simulink model "BMS_PIL_Wrapper"  (R2025b)
settings: Solver=ode3  StartTime=0.0  StopTime=20  FixedStep=.001  MaxStep=.01  RelTol=1e-3  EnableMultiTasking=on
PreLoadFcn:
  | setup_pil;
InitFcn:
  | battery_init;
  | Full_Charge_Volt=4.2; % unit volts
  | Cutoff_Volt=3; % unit volts
  | Delta=.02;
  | ContactorTime=20;
  | ContactorTimeOut=100;
  | High_TempLim=333;
  | Low_TempLim=253;
  | Sensor_Fault_Treshold=.02;
  | CurrentTimeout=1;
  | Allowed_Delta=.04;
  | Bal_On_Time=30;
  | Bal_Off_Time=5;
  | BalNotAct_Time=10;
values from neighbouring files (symbols this model uses):
  Cell_Num = 12    [From_Plant_IC.m]
  Fly_Cycle_Current = [ ... (first row only)    [battery_init.m]
undefined symbols (not defined in the file or in its folder): SRE
libraries: fl_lib x69, nesl_utility x54, ee_lib x12, batteryecm_lib x12, simulink x5, BatteryCurrentManagement x1
(part 4 of 4)

== stateflow chart BMS_PIL_Wrapper/Test Sequence ==
  state Flying
    State_Required=SRE.Charge
  state step_2
  (default) -> Flying
  Flying -> step_2
  data: State_Required output

== stateflow chart BMS_PIL_Wrapper/FC/Chart ==
  state Needed_Action
    if Fault_Level == 4
    Drone_Mode = 4;
    Motor_Command = 0;
    elseif Fault_Level == 3
    Drone_Mode = 3;
    Motor_Command = 0.3;
    elseif Fault_Level == 2
    Drone_Mode = 2;
    Motor_Command = 0.6;
    elseif Fault_Level == 1
    Drone_Mode = 1;
    Motor_Command = 1.0;
    else
    Drone_Mode = 0;
    Motor_Command = 1.0;
    end
  (default) -> Needed_Action
  data: Drone_Mode output; Motor_Command output; Fault_Level input
